simulink model "kalman_filter_tuning"  (R2021a)
settings: Solver=VariableStepAuto  StartTime=0.0  StopTime=15  RelTol=1e-3
values from neighbouring files (symbols this model uses):
  A_a_dis = [1  -0.0479044950468; 0  1]    [RSdata_Kalman.mat]
  A_e_dis = [1  0.0479044950468; 0  1]    [RSdata_Kalman.mat]
  A_t_dis = [1  0.00488821378028; 0  1]    [RSdata_Kalman.mat]
  B_a_dis = [-0.000119761237617 0.005]    [RSdata_Kalman.mat]
  B_e_dis = [0.000119761237617 0.005]    [RSdata_Kalman.mat]
  B_t_dis = [1.22205344507e-05 0.005]    [RSdata_Kalman.mat]
  C_a_dis = [1  0; 0  1]    [RSdata_Kalman.mat]
  C_e_dis = [1  0; 0  1]    [RSdata_Kalman.mat]
  C_t_dis = [1 0]    [RSdata_Kalman.mat]
  R_t = 0.00678306479724    [RSdata_Kalman.mat]
undefined symbols (not defined in the file or in its folder): Discrete, Time
libraries: ctrlSharedLib x3
settings Model: Creator=tomwh  LastModifiedBy=tomwh

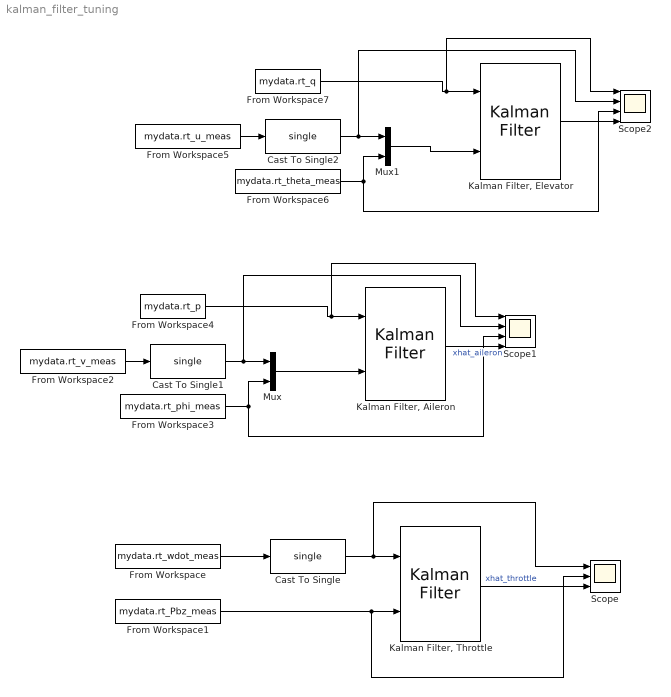
== system kalman_filter_tuning ==
  Cast To Single : DataTypeConversion  OutDataTypeStr=single
  Cast To Single1 : DataTypeConversion  OutDataTypeStr=single
  Cast To Single2 : DataTypeConversion  OutDataTypeStr=single
  From Workspace : FromWorkspace  VariableName=mydata.rt_wdot_meas  SampleTime=1/200
  From Workspace1 : FromWorkspace  VariableName=mydata.rt_Pbz_meas  SampleTime=1/200
  From Workspace2 : FromWorkspace  VariableName=mydata.rt_v_meas  SampleTime=1/200
  From Workspace3 : FromWorkspace  VariableName=mydata.rt_phi_meas  SampleTime=1/200
  From Workspace4 : FromWorkspace  VariableName=mydata.rt_p  SampleTime=1/200
  From Workspace5 : FromWorkspace  VariableName=mydata.rt_u_meas  SampleTime=1/200
  From Workspace6 : FromWorkspace  VariableName=mydata.rt_theta_meas  SampleTime=1/200
  From Workspace7 : FromWorkspace  VariableName=mydata.rt_q  SampleTime=1/200
  "Kalman Filter, Aileron" : ctrlSharedLib/Kalman Filter  TimeDomain=Discrete-Time  UseCurrentEstimator=on  ModelSource=Individual A, B, C, D matrices  ModelSourceVariable=ss(0.95,1,1,0,1)  A=A_a_dis  B=B_a_dis  C=C_a_dis  D=0  NumberOfStates=1  NumberOfInputs=1  NumberOfOutputs=1  InitialEstimateSource=Dialog  X0=0  P0=10  UseK=off  UseGH=off  NumberOfProcessNoiseInputs=1  G=1  TimeInvariantG=on  H=0  TimeInvariantH=on  Q=Q_a_dis  TimeInvariantQ=on  R=[1 0; 0 1/25]  TimeInvariantR=on  N=0  TimeInvariantN=on  AddInputPort=on  AddEnablePort=off  OutputEstimatedY=off  OutputP=off  Ts=1/200
  "Kalman Filter, Elevator" : ctrlSharedLib/Kalman Filter  TimeDomain=Discrete-Time  UseCurrentEstimator=on  ModelSource=Individual A, B, C, D matrices  ModelSourceVariable=ss(0.95,1,1,0,1)  A=A_e_dis  B=B_e_dis  C=C_e_dis  D=0  NumberOfStates=1  NumberOfInputs=1  NumberOfOutputs=1  InitialEstimateSource=Dialog  X0=0  P0=10  UseK=off  UseGH=off  NumberOfProcessNoiseInputs=1  G=1  TimeInvariantG=on  H=0  TimeInvariantH=on  Q=Q_e_dis  TimeInvariantQ=on  R=[1/100 0; 0 1/25]  TimeInvariantR=on  N=0  TimeInvariantN=on  AddInputPort=on  AddEnablePort=off  OutputEstimatedY=off  OutputP=off  Ts=1/200
  "Kalman Filter, Throttle" : ctrlSharedLib/Kalman Filter  TimeDomain=Discrete-Time  UseCurrentEstimator=on  ModelSource=Individual A, B, C, D matrices  ModelSourceVariable=ss(0.95,1,1,0,1)  A=A_t_dis  B=B_t_dis  C=C_t_dis  D=0  NumberOfStates=1  NumberOfInputs=1  NumberOfOutputs=1  InitialEstimateSource=Dialog  X0=0  P0=10  UseK=off  UseGH=off  NumberOfProcessNoiseInputs=1  G=1  TimeInvariantG=on  H=0  TimeInvariantH=on  Q=Q_t_dis  TimeInvariantQ=on  R=R_t  TimeInvariantR=on  N=0  TimeInvariantN=on  AddInputPort=on  AddEnablePort=off  OutputEstimatedY=off  OutputP=off  Ts=1/200
  Mux : Mux  Inputs=2
  Mux1 : Mux  Inputs=2
  Scope : Scope  NumInputPorts=3
  Scope1 : Scope  NumInputPorts=4
  Scope2 : Scope  NumInputPorts=4
  wires:
  From Workspace1/1 -> Scope/2, "Kalman Filter, Throttle"/2
  "Kalman Filter, Throttle"/1 -> Scope/3  "xhat_throttle"
  From Workspace/1 -> Cast To Single/1
  Cast To Single/1 -> Scope/1, "Kalman Filter, Throttle"/1
  From Workspace4/1 -> Scope1/1, "Kalman Filter, Aileron"/1
  Mux/1 -> "Kalman Filter, Aileron"/2
  From Workspace3/1 -> Mux/2, Scope1/3
  "Kalman Filter, Aileron"/1 -> Scope1/4  "xhat_aileron"
  From Workspace2/1 -> Cast To Single1/1
  Cast To Single1/1 -> Scope1/2, Mux/1
  "Kalman Filter, Elevator"/1 -> Scope2/4
  Cast To Single2/1 -> Scope2/2, Mux1/1
  From Workspace5/1 -> Cast To Single2/1
  From Workspace6/1 -> Mux1/2, Scope2/3
  From Workspace7/1 -> "Kalman Filter, Elevator"/1, Scope2/1
  Mux1/1 -> "Kalman Filter, Elevator"/2
